simulink model "ComparativoModeloLinear"  (R2021a)
settings: Solver=VariableStepAuto  StartTime=0.0  StopTime=500  RelTol=1e-3
settings Model: Creator=Usuario  LastModifiedBy=Usuario

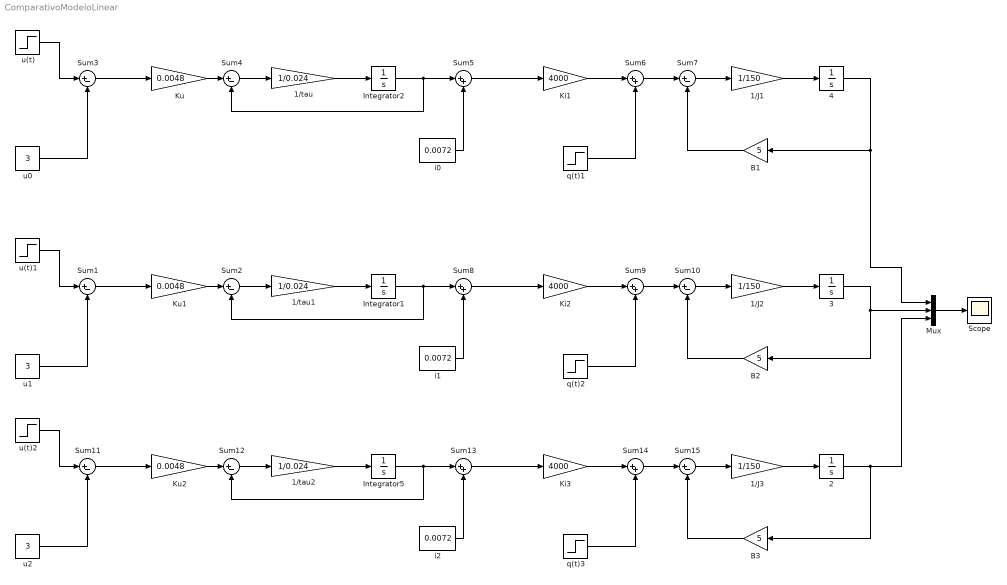
== system ComparativoModeloLinear ==
  1/J1 : Gain  Gain=1/150
  1/J2 : Gain  Gain=1/150
  1/J3 : Gain  Gain=1/150
  1/tau : Gain  Gain=1/0.024
  1/tau1 : Gain  Gain=1/0.024
  1/tau2 : Gain  Gain=1/0.024
  2 : Integrator
  3 : Integrator
  4 : Integrator
  B1 : Gain  Gain=5
  B2 : Gain  Gain=5
  B3 : Gain  Gain=5
  Integrator1 : Integrator
  Integrator2 : Integrator
  Integrator5 : Integrator
  Ki1 : Gain  Gain=4000
  Ki2 : Gain  Gain=4000
  Ki3 : Gain  Gain=4000
  Ku : Gain  Gain=0.0048
  Ku1 : Gain  Gain=0.0048
  Ku2 : Gain  Gain=0.0048
  Mux : Mux  Inputs=3
  Scope : Scope
  Sum{1..4,7,10..12,15} (9 alike) : Sum  Inputs=|+-
  Sum{5..6,8..9,13..14} (6 alike) : Sum  Inputs=|++
  i0 : Constant  Value=0.0072
  i1 : Constant  Value=0.0072
  i2 : Constant  Value=0.0072
  q(t)1 : Step  Time=250  After=5  SampleTime=0
  q(t)2 : Step  Time=250  After=0  SampleTime=0
  q(t)3 : Step  Time=250  After=-5  SampleTime=0
  u(t) : Step  Time=250  Before=3  After=3  SampleTime=0
  u(t)1 : Step  Time=250  Before=3  After=3  SampleTime=0
  u(t)2 : Step  Time=250  Before=3  After=3  SampleTime=0
  u0 : Constant  Value=3
  u1 : Constant  Value=3
  u2 : Constant  Value=3
  wires:
  u(t)/1 -> Sum3/1
  4/1 -> Mux/1, B1/1
  i0/1 -> Sum5/2
  Ki1/1 -> Sum6/1
  q(t)1/1 -> Sum6/2
  1/J1/1 -> 4/1
  Sum6/1 -> Sum7/1
  Ku/1 -> Sum4/1
  Sum4/1 -> 1/tau/1
  Sum5/1 -> Ki1/1
  u0/1 -> Sum3/2
  1/tau/1 -> Integrator2/1
  B1/1 -> Sum7/2
  Sum7/1 -> 1/J1/1
  Integrator2/1 -> Sum4/2, Sum5/1
  Sum3/1 -> Ku/1
  Mux/1 -> Scope/1
  Sum9/1 -> Sum10/1
  Ki2/1 -> Sum9/1
  1/J2/1 -> 3/1
  q(t)2/1 -> Sum9/2
  i1/1 -> Sum8/2
  3/1 -> B2/1, Mux/2
  u(t)1/1 -> Sum1/1
  Sum1/1 -> Ku1/1
  Sum8/1 -> Ki2/1
  Sum2/1 -> 1/tau1/1
  Sum10/1 -> 1/J2/1
  B2/1 -> Sum10/2
  1/tau1/1 -> Integrator1/1
  u1/1 -> Sum1/2
  Ku1/1 -> Sum2/1
  Integrator1/1 -> Sum2/2, Sum8/1
  Sum14/1 -> Sum15/1
  Ki3/1 -> Sum14/1
  1/J3/1 -> 2/1
  q(t)3/1 -> Sum14/2
  i2/1 -> Sum13/2
  2/1 -> Mux/3, B3/1
  u(t)2/1 -> Sum11/1
  Sum11/1 -> Ku2/1
  Sum13/1 -> Ki3/1
  Sum12/1 -> 1/tau2/1
  Sum15/1 -> 1/J3/1
  B3/1 -> Sum15/2
  1/tau2/1 -> Integrator5/1
  u2/1 -> Sum11/2
  Ku2/1 -> Sum12/1
  Integrator5/1 -> Sum12/2, Sum13/1
